simulink model "OK"  (R2021a)
settings: Solver=VariableStepAuto  StartTime=0.0  StopTime=10.0  RelTol=1e-3
settings Model: Creator=ritav  LastModifiedBy=ritav

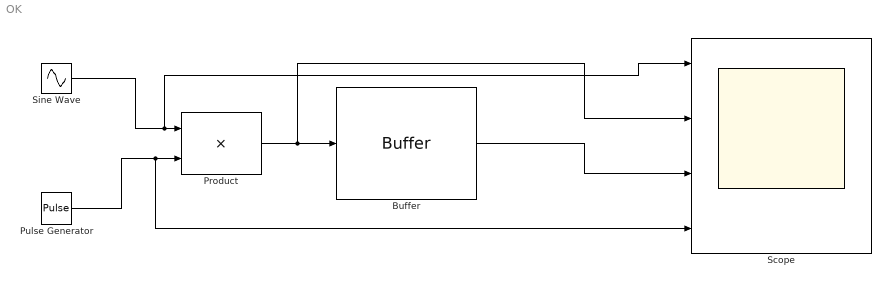
== system OK ==
  Buffer : Buffer  OutputFrames=off
  Product : Product
  Pulse Generator : DiscretePulseGenerator  PulseType=Time based  Period=10  PulseWidth=5
  Scope : Scope  NumInputPorts=4
  Sine Wave : Sin  Frequency=5  SampleTime=0.001
  wires:
  Pulse Generator/1 -> Scope/4, Product/2
  Sine Wave/1 -> Scope/1, Product/1
  Buffer/1 -> Scope/3
  Product/1 -> Scope/2, Buffer/1
